simulink model "Week1problem8"  (R2020b)
settings: Solver=VariableStepAuto  StartTime=0.0  StopTime=10.0  RelTol=1e-3
settings Model: Creator=HP  LastModifiedBy=HP

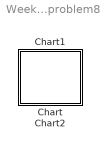
== system Week1problem8 ==
  Chart : Stateflow chart  TreatAsAtomicUnit=on
  Chart1 : Stateflow chart  TreatAsAtomicUnit=on
  Chart2 : Stateflow chart  TreatAsAtomicUnit=on

== stateflow chart Week1problem8/Chart1 ==

== stateflow chart Week1problem8/Chart2 ==
  state LiftOperation
    entry:
    status=0;
    state LiftFunctionOn
      (history)
      state GroundFloor
        entry:
        status=1;
        during:
        CurrentFloor=0;
        FloorCheck(CurrentFloor);
        exit:
        status=0;
      state FirstFloor
        entry:
        status=1;
        during:
        CurrentFloor=1;
        FloorCheck(CurrentFloor);
        exit:
        status=0;
      state SecondFloor
        entry:
        status=1;
        during:
        CurrentFloor=2;
        FloorCheck(CurrentFloor);
        exit:
        status=0;
        after(1,sec);
      state ThirdFloor
        entry:
        status=1;
        during:
        CurrentFloor=3;
        FloorCheck(CurrentFloor);
        exit:
        status=0;
        after(1,sec);
      state FourthFloor
        entry:
        status=1
        during:
        CurrentFloor=4;
        FloorCheck(CurrentFloor);
        exit:
        status=0;
      state FifthFloor
        entry:
        status=1;
        during:
        CurrentFloor=5;
        FloorCheck(CurrentFloor);
        exit:
        status=0;
      (default) -> GroundFloor
      GroundFloor -> FirstFloor : up
      FirstFloor -> GroundFloor [order 2] : down
      FirstFloor -> SecondFloor [order 1] : up
      SecondFloor -> FirstFloor [order 2] : down
      SecondFloor -> ThirdFloor [order 1] : up
      ThirdFloor -> SecondFloor [order 2] : down
      ThirdFloor -> FourthFloor [order 1] : up
      FourthFloor -> ThirdFloor [order 1] : down
      FourthFloor -> FifthFloor [order 2] : up
      FifthFloor -> FourthFloor : down
    state LiftFunctionOff
      en:
      status=0;
    (default) -> LiftFunctionOn
    LiftFunctionOff -> LiftFunctionOn : [signal==0]
    LiftFunctionOn -> LiftFunctionOff : [signal==1]
  state Alarm
    during:
    AlarmStatus = fire;
    FireStatusCheck(AlarmStatus);
  state FireStatusCheck(AlarmSt) [function]
    (default) -> (junction 43)
    (junction 43) -> (junction 40) [order 1] : [AlarmSt ==0]
    (junction 43) -> (junction 32) [order 2] : {signal=1;}
    (junction 40) -> (junction 41) : {signal=0;}
    (junction 41) -> (junction 32)
    (junction 32) -> (junction 31)
  state FloorCheck(Floor) [function]
    (default) -> (junction 42) : [FloorSelect<Floor]{
        | send(down);
        | disp('LiftMovingDown');}
    (junction 42) -> (junction 29)
    (junction 29) -> ?
  (default) -> LiftOperation
  data: AlarmSt function_input; Floor function_input

== stateflow chart Week1problem8/Chart ==
